simulink model "SE"  (R2019b)
settings: Solver=FixedStepDiscrete  StartTime=0.0  StopTime=stop_time  RelTol=1e-3
InitFcn:
  | sm_callback_init
StopFcn:
  | sm_callback_stop
values from neighbouring files (symbols this model uses):
  mp = sm_stop_verify(mp)    [sm_callback_stop.m]
libraries: hdlsllib x6, simulink x3
settings Model: Creator=Ross  LastModifiedBy=wickh
settings DataIOCC: ReturnWorkspaceOutputs=off
settings OptimizationCC: BlockReduction=off  ConditionallyExecuteInputs=off  DefaultParameterBehavior=Inlined
settings DebuggingCC: ReadBeforeWriteMsg=DisableAll  WriteAfterWriteMsg=DisableAll  WriteAfterReadMsg=DisableAll  AlgebraicLoopMsg=error  MultiTaskDSMMsg=none  SingleTaskRateTransMsg=error  PregeneratedLibrarySubsystemCodeDiagnostic=none  ArithmeticOperatorsInVariantConditions=warning
settings HardwareCC: ProdBitPerPointer=32  ProdBitPerSizeT=32  ProdBitPerPtrDiffT=32  ProdLargestAtomicFloat=None  ProdIntDivRoundTo=Undefined  ProdEndianess=Unspecified  ProdWordSize=32  ProdHWDeviceType=ASIC/FPGA->ASIC/FPGA  TargetBitPerPointer=64  TargetBitPerSizeT=64  TargetBitPerPtrDiffT=64  TargetLongLongMode=on  TargetIntDivRoundTo=Zero  TargetEndianess=LittleEndian  TargetWordSize=64  TargetHWDeviceType=Custom Processor->MATLAB Host Computer  ProdEqTarget=off
settings ModelReferenceCC: UpdateModelReferenceTargets=IfOutOfDate
settings SFSimCC: SFSimEcho=off  SimUseLocalCustomCode=off  CustomCodeUndefinedFunction=UseInterfaceOnly
settings RTWCC: RTWUseLocalCustomCode=off

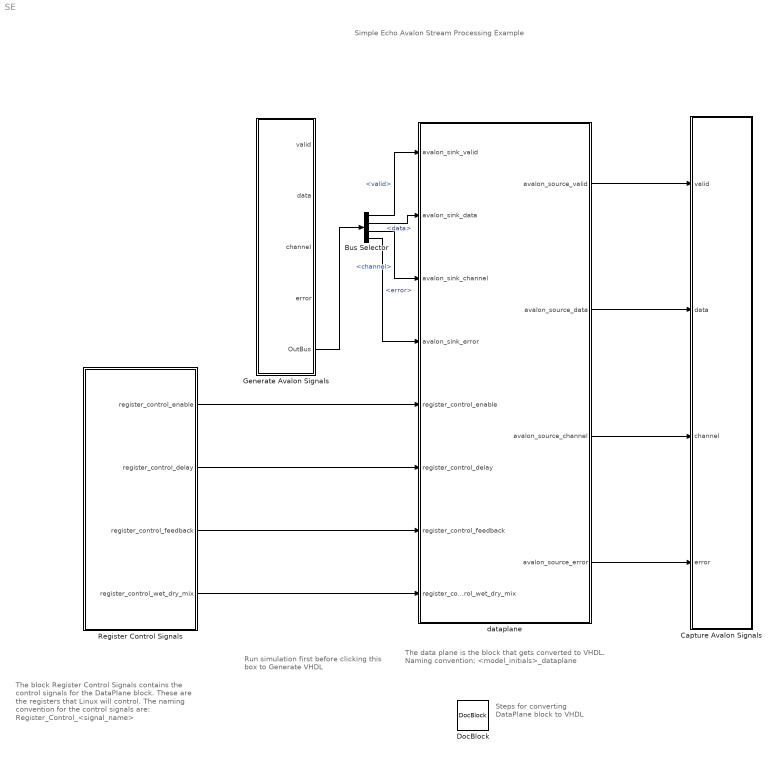
== system SE ==
  note: The data plane is the block that gets converted to VHDL. Naming convention: <model_initials>_dataplane
  note: Steps for converting
      | DataPlane block
      | to VHDL
  note: Simple Echo
      | Avalon Stream Processing Example
  note: Run simulation first
      | before clicking this box to
      | Generate VHDL
  note: The block Register Control Signals contains
      | the control signals for the DataPlane block.
      | These are the registers that Linux will control.
      | The naming convention for the control
      | signals are:  Register_Control_<signal_name>
  Bus Selector : BusSelector  OutputSignals=Avalon.valid,Avalon.data,Avalon.channel,Avalon.error
  Capture Avalon Signals : Subsystem
  DocBlock : simulink/Model-Wide Utilities/DocBlock  DocumentType=HTML
  Generate Avalon Signals : Subsystem
  Register Control Signals : Subsystem
  dataplane : Subsystem  TreatAsAtomicUnit=on
  wires:
  dataplane/2(avalon_source_data) -> Capture Avalon Signals/2(data)
  dataplane/1(avalon_source_valid) -> Capture Avalon Signals/1(valid)
  dataplane/3(avalon_source_channel) -> Capture Avalon Signals/3(channel)
  dataplane/4(avalon_source_error) -> Capture Avalon Signals/4(error)
  Register Control Signals/2(register_control_delay) -> dataplane/6(register_control_delay)
  Register Control Signals/1(register_control_enable) -> dataplane/5(register_control_enable)
  Register Control Signals/4(register_control_wet_dry_mix) -> dataplane/8(register_control_wet_dry_mix)
  Register Control Signals/3(register_control_feedback) -> dataplane/7(register_control_feedback)
  Generate Avalon Signals/5(OutBus) -> Bus Selector/1
  Bus Selector/1 -> dataplane/1(avalon_sink_valid)  "<valid>"
  Bus Selector/2 -> dataplane/2(avalon_sink_data)  "<data>"
  Bus Selector/3 -> dataplane/3(avalon_sink_channel)  "<channel>"
  Bus Selector/4 -> dataplane/4(avalon_sink_error)  "<error>"

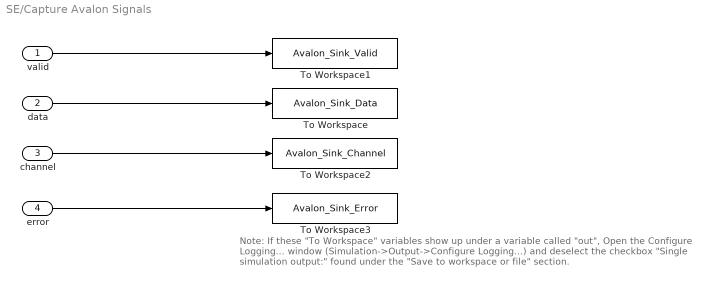
== system SE/Capture Avalon Signals ==
  note: Note:  If these "To Workspace" variables show up under a variable called "out",
      | Open the Configure Logging... window (Simulation->Output->Configure Logging...)
      | and deselect the checkbox "Single simulation output:" found under the "Save to workspace or file" section.
  valid : Inport
  data : Inport  Port=2
  channel : Inport  Port=3
  error : Inport  Port=4
  To Workspace : ToWorkspace  VariableName=Avalon_Sink_Data  SaveFormat=Timeseries  SampleTime=-1
  To Workspace1 : ToWorkspace  VariableName=Avalon_Sink_Valid  SaveFormat=Timeseries  SampleTime=-1
  To Workspace2 : ToWorkspace  VariableName=Avalon_Sink_Channel  SaveFormat=Timeseries  SampleTime=-1
  To Workspace3 : ToWorkspace  VariableName=Avalon_Sink_Error  SaveFormat=Timeseries  SampleTime=-1
  wires:
  data/1 -> To Workspace/1
  valid/1 -> To Workspace1/1
  error/1 -> To Workspace3/1
  channel/1 -> To Workspace2/1

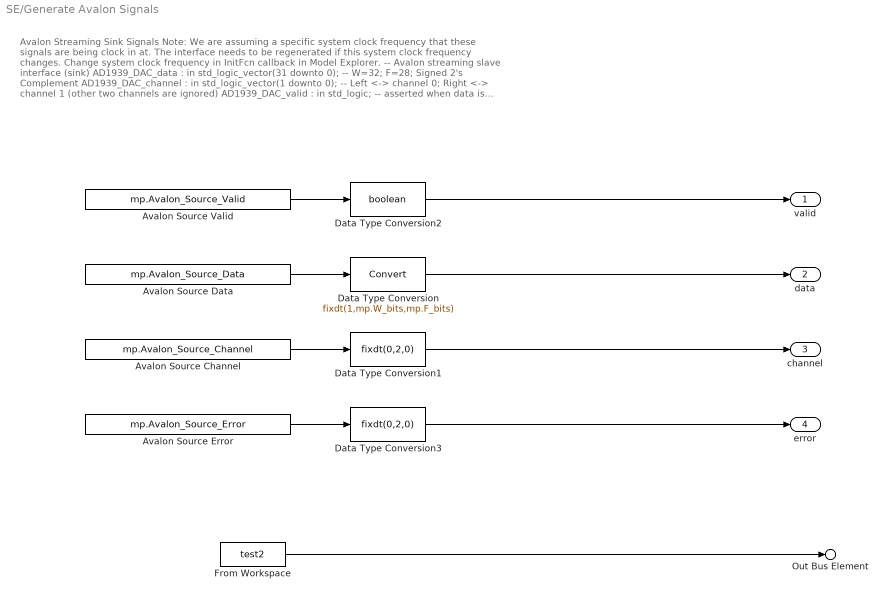
== system SE/Generate Avalon Signals ==
  note: Avalon Streaming Sink Signals
      | Note: We are assuming a specific system clock frequency that these signals are being clock in at.
      | The interface needs to be regenerated if this system clock frequency changes. Change system clock frequency in InitFcn callback in Model Explorer.
      |
      | -- Avalon streaming slave interface (sink)
      | AD1939_DAC_data : in std_logic_vector(31 downto 0); -- W=32; F=28; Signed 2's Complement
      | AD1939_DAC_channel : in std_logic_vector(1 downto 0); -- Left <-> channel 0; Right <-> channel 1 (other two channels are ignored)
      | AD1939_DAC_valid : in std_logic; -- asserted when data is valid
      | AD1939_DAC_error : in std_logic_vector(1 downto 0) -- error channel is ignored, assumed to be error free at this point
      |
      | For more information on the data-channel-valid protocol, s ee chapter 5 in Intel's Avalon Interfaced Specification (p. 40) at https://www.intel.com/content/dam/www/programmable/us/en/pdfs/literature/manual/mnl_avalon_spec.pdf
  Avalon Source Channel : FromWorkspace  VariableName=mp.Avalon_Source_Channel  OutDataTypeStr=double  SampleTime=mp.Ts_system
  "Avalon Source Data " : FromWorkspace  VariableName=mp.Avalon_Source_Data  OutDataTypeStr=double  SampleTime=mp.Ts_system
  Avalon Source Error : FromWorkspace  VariableName=mp.Avalon_Source_Error  OutDataTypeStr=double  SampleTime=mp.Ts_system
  Avalon Source Valid : FromWorkspace  VariableName=mp.Avalon_Source_Valid  OutDataTypeStr=double  SampleTime=mp.Ts_system
  Data Type Conversion : DataTypeConversion  OutDataTypeStr=fixdt(1,mp.W_bits,mp.F_bits)
  Data Type Conversion1 : DataTypeConversion  OutDataTypeStr=fixdt(0,2,0)
  Data Type Conversion2 : DataTypeConversion  OutDataTypeStr=boolean
  Data Type Conversion3 : DataTypeConversion  OutDataTypeStr=fixdt(0,2,0)
  From Workspace : FromWorkspace  VariableName=test2  OutDataTypeStr=Bus: AvalonBus  SampleTime=0
  valid : Outport  VectorParamsAs1DForOutWhenUnconnected=off
  data : Outport  Port=2  VectorParamsAs1DForOutWhenUnconnected=off
  channel : Outport  Port=3  VectorParamsAs1DForOutWhenUnconnected=off
  error : Outport  Port=4  VectorParamsAs1DForOutWhenUnconnected=off
  Out Bus Element : Outport  Port=5  PortName=OutBus  Element=Avalon
  wires:
  Data Type Conversion1/1 -> channel/1
  Data Type Conversion2/1 -> valid/1
  Avalon Source Error/1 -> Data Type Conversion3/1
  Data Type Conversion/1 -> data/1
  Avalon Source Valid/1 -> Data Type Conversion2/1
  Data Type Conversion3/1 -> error/1
  Avalon Source Channel/1 -> Data Type Conversion1/1
  "Avalon Source Data "/1 -> Data Type Conversion/1
  From Workspace/1 -> Out Bus Element/1

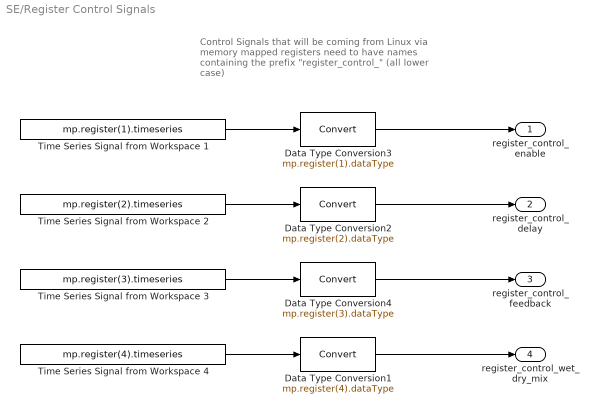
== system SE/Register Control Signals ==
  note: Control Signals that will be coming from Linux via
      | memory mapped registers need to have names
      | containing the prefix "register_control_"
      | (all lower case)
  Data Type Conversion1 : DataTypeConversion  OutDataTypeStr=mp.register(4).dataType
  Data Type Conversion2 : DataTypeConversion  OutDataTypeStr=mp.register(2).dataType
  Data Type Conversion3 : DataTypeConversion  OutDataTypeStr=mp.register(1).dataType
  Data Type Conversion4 : DataTypeConversion  OutDataTypeStr=mp.register(3).dataType
  Time Series Signal from Workspace 1 : FromWorkspace  VariableName=mp.register(1).timeseries  OutDataTypeStr=double  SampleTime=mp.Ts_system
  Time Series Signal from Workspace 2 : FromWorkspace  VariableName=mp.register(2).timeseries  OutDataTypeStr=double  SampleTime=mp.Ts_system
  Time Series Signal from Workspace 3 : FromWorkspace  VariableName=mp.register(3).timeseries  OutDataTypeStr=double  SampleTime=mp.Ts_system
  Time Series Signal from Workspace 4 : FromWorkspace  VariableName=mp.register(4).timeseries  OutDataTypeStr=double  SampleTime=mp.Ts_system
  register_control_enable : Outport  VectorParamsAs1DForOutWhenUnconnected=off
  register_control_delay : Outport  Port=2  VectorParamsAs1DForOutWhenUnconnected=off
  register_control_feedback : Outport  Port=3  VectorParamsAs1DForOutWhenUnconnected=off
  register_control_wet_dry_mix : Outport  Port=4  VectorParamsAs1DForOutWhenUnconnected=off
  wires:
  Time Series Signal from Workspace 2/1 -> Data Type Conversion2/1
  Data Type Conversion2/1 -> register_control_delay/1
  Time Series Signal from Workspace 1/1 -> Data Type Conversion3/1
  Data Type Conversion3/1 -> register_control_enable/1
  Time Series Signal from Workspace 4/1 -> Data Type Conversion1/1
  Data Type Conversion1/1 -> register_control_wet_dry_mix/1
  Data Type Conversion4/1 -> register_control_feedback/1
  Time Series Signal from Workspace 3/1 -> Data Type Conversion4/1

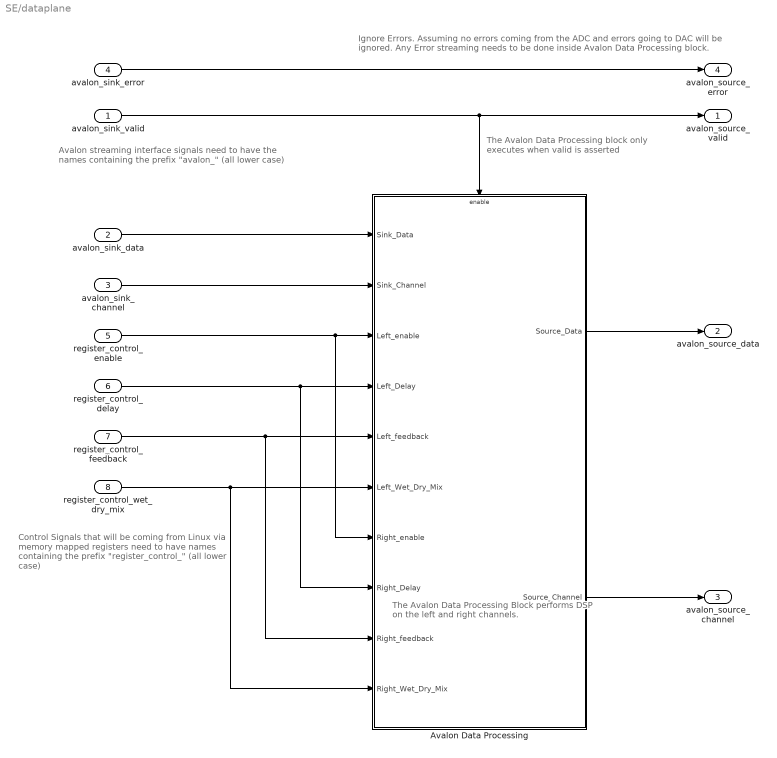
== system SE/dataplane ==
  note: Control Signals that will be coming from Linux via
      | memory mapped registers need to have names
      | containing the prefix "register_control_"
      | (all lower case)
  note: The Avalon Data Processing Block
      | performs DSP on the left and right channels.
  note: The Avalon Data Processing block
      | only executes when valid is asserted
  note: Ignore Errors.
      | Assuming no errors coming from the ADC and errors going to DAC will be ignored.
      | Any Error streaming needs to be done inside Avalon Data Processing block.
  note: Avalon streaming interface signals need to have the
      | names containing the prefix "avalon_"
      | (all lower case)
  avalon_sink_valid : Inport
  avalon_sink_data : Inport  Port=2
  avalon_sink_channel : Inport  Port=3
  avalon_sink_error : Inport  Port=4
  register_control_enable : Inport  Port=5
  register_control_delay : Inport  Port=6
  register_control_feedback : Inport  Port=7
  register_control_wet_dry_mix : Inport  Port=8
  Avalon Data Processing : Subsystem  TreatAsAtomicUnit=on
  avalon_source_valid : Outport  VectorParamsAs1DForOutWhenUnconnected=off
  avalon_source_data : Outport  Port=2  VectorParamsAs1DForOutWhenUnconnected=off
  avalon_source_channel : Outport  Port=3  VectorParamsAs1DForOutWhenUnconnected=off
  avalon_source_error : Outport  Port=4  VectorParamsAs1DForOutWhenUnconnected=off
  wires:
  avalon_sink_channel/1 -> Avalon Data Processing/2(Sink_Channel)
  avalon_sink_error/1 -> avalon_source_error/1
  Avalon Data Processing/1(Source_Data) -> avalon_source_data/1
  avalon_sink_valid/1 -> avalon_source_valid/1, Avalon Data Processing/Enable
  avalon_sink_data/1 -> Avalon Data Processing/1(Sink_Data)
  Avalon Data Processing/2(Source_Channel) -> avalon_source_channel/1
  register_control_delay/1 -> Avalon Data Processing/8(Right_Delay), Avalon Data Processing/4(Left_Delay)
  register_control_enable/1 -> Avalon Data Processing/7(Right_enable), Avalon Data Processing/3(Left_enable)
  register_control_wet_dry_mix/1 -> Avalon Data Processing/6(Left_Wet_Dry_Mix), Avalon Data Processing/10(Right_Wet_Dry_Mix)
  register_control_feedback/1 -> Avalon Data Processing/9(Right_feedback), Avalon Data Processing/5(Left_feedback)

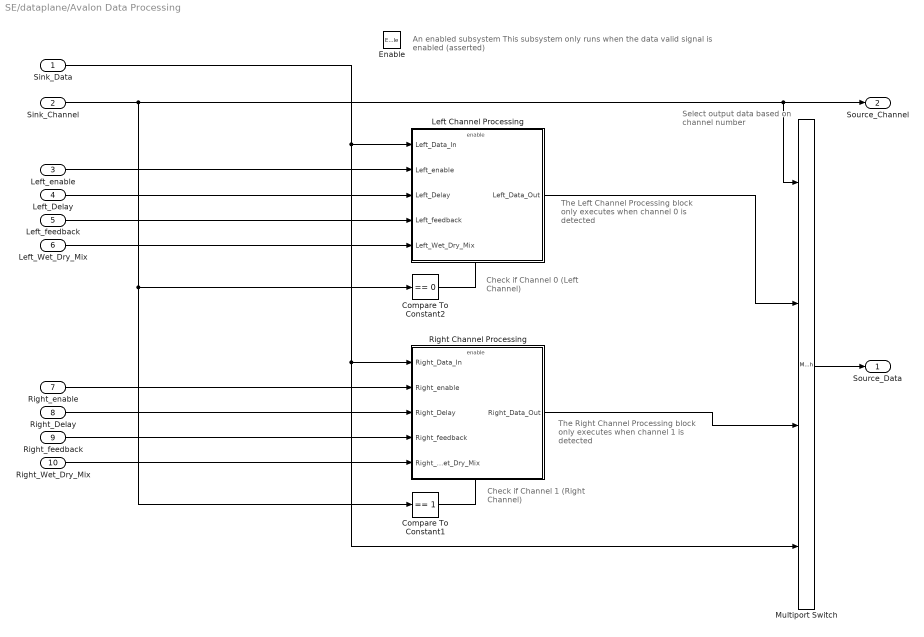
== system SE/dataplane/Avalon Data Processing ==
  note: Select output data
      | based on channel number
  note: Check if Channel 0
      | (Left Channel)
  note: The Left Channel Processing block
      | only executes when channel 0
      | is detected
  note: The Right Channel Processing block
      | only executes when channel 1
      | is detected
  note: Check if Channel 1
      | (Right Channel)
  note: An enabled subsystem
      | This subsystem only runs when the data valid signal is enabled (asserted)
  Sink_Data : Inport
  Sink_Channel : Inport  Port=2
  Left_enable : Inport  Port=3
  Left_Delay : Inport  Port=4
  Left_feedback : Inport  Port=5
  Left_Wet_Dry_Mix : Inport  Port=6
  Right_enable : Inport  Port=7
  Right_Delay : Inport  Port=8
  Right_feedback : Inport  Port=9
  Right_Wet_Dry_Mix : Inport  Port=10
  Enable : EnablePort
  Compare To Constant1 : simulink/Logic and Bit Operations/Compare To Constant  relop===  const=1  OutDataTypeStr=boolean
  Compare To Constant2 : simulink/Logic and Bit Operations/Compare To Constant  relop===  const=0  OutDataTypeStr=boolean
  Left Channel Processing : Subsystem  TreatAsAtomicUnit=on
  Multiport Switch : MultiPortSwitch  DataPortOrder=Zero-based contiguous  zeroidx=on
  Right Channel Processing : Subsystem  TreatAsAtomicUnit=on
  Source_Data : Outport  InitialOutput=0  VectorParamsAs1DForOutWhenUnconnected=off
  Source_Channel : Outport  Port=2  InitialOutput=0  VectorParamsAs1DForOutWhenUnconnected=off
  wires:
  Sink_Channel/1 -> Compare To Constant1/1, Compare To Constant2/1, Source_Channel/1, Multiport Switch/1
  Compare To Constant2/1 -> Left Channel Processing/Enable
  Compare To Constant1/1 -> Right Channel Processing/Enable
  Sink_Data/1 -> Multiport Switch/4, Right Channel Processing/1(Right_Data_In), Left Channel Processing/1(Left_Data_In)
  Left Channel Processing/1("Left_Data_Out ") -> Multiport Switch/2
  Right Channel Processing/1("Right_Data_Out ") -> Multiport Switch/3
  Multiport Switch/1 -> Source_Data/1
  Left_Delay/1 -> Left Channel Processing/3(Left_Delay)
  Right_Delay/1 -> Right Channel Processing/3(Right_Delay)
  Left_enable/1 -> Left Channel Processing/2(Left_enable)
  Right_enable/1 -> Right Channel Processing/2(Right_enable)
  Left_Wet_Dry_Mix/1 -> Left Channel Processing/5(Left_Wet_Dry_Mix)
  Right_Wet_Dry_Mix/1 -> Right Channel Processing/5(Right_Wet_Dry_Mix)
  Left_feedback/1 -> Left Channel Processing/4(Left_feedback)
  Right_feedback/1 -> Right Channel Processing/4(Right_feedback)

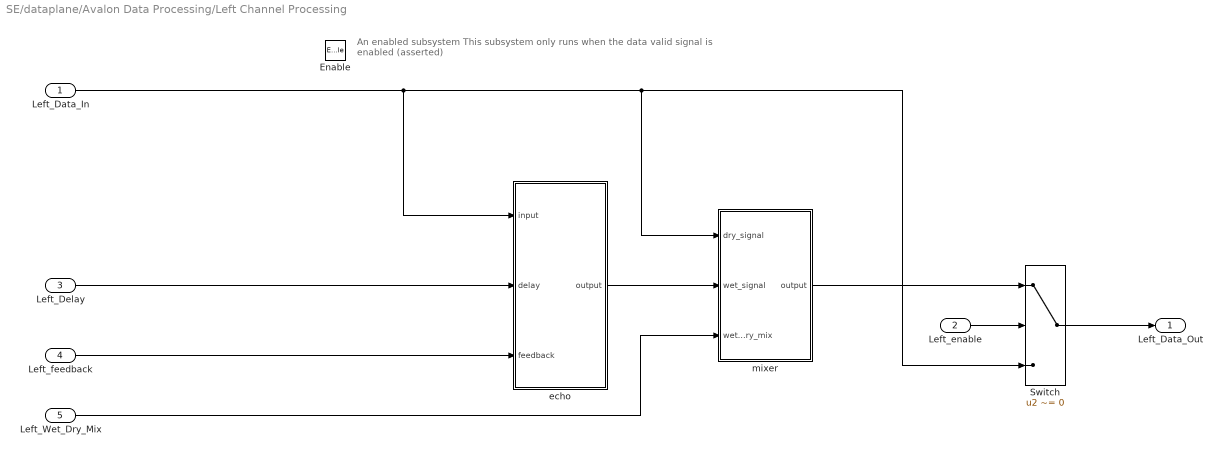
== system SE/dataplane/Avalon Data Processing/Left Channel Processing ==
  note: An enabled subsystem
      | This subsystem only runs when the data valid signal is enabled (asserted)
  Left_Data_In : Inport
  Left_enable : Inport  Port=2
  Left_Delay : Inport  Port=3
  Left_feedback : Inport  Port=4
  Left_Wet_Dry_Mix : Inport  Port=5
  Enable : EnablePort
  Switch : Switch  Criteria=u2 ~= 0
  echo : Subsystem
  mixer : Subsystem
  "Left_Data_Out " : Outport  InitialOutput=0  VectorParamsAs1DForOutWhenUnconnected=off
  wires:
  Left_Data_In/1 -> echo/1(input), mixer/1(dry_signal), Switch/3
  Switch/1 -> "Left_Data_Out "/1
  Left_enable/1 -> Switch/2
  echo/1(output) -> mixer/2(wet_signal)
  Left_Wet_Dry_Mix/1 -> mixer/3(wet_dry_mix)
  Left_Delay/1 -> echo/2(delay)
  Left_feedback/1 -> echo/3(feedback)
  mixer/1(output) -> Switch/1

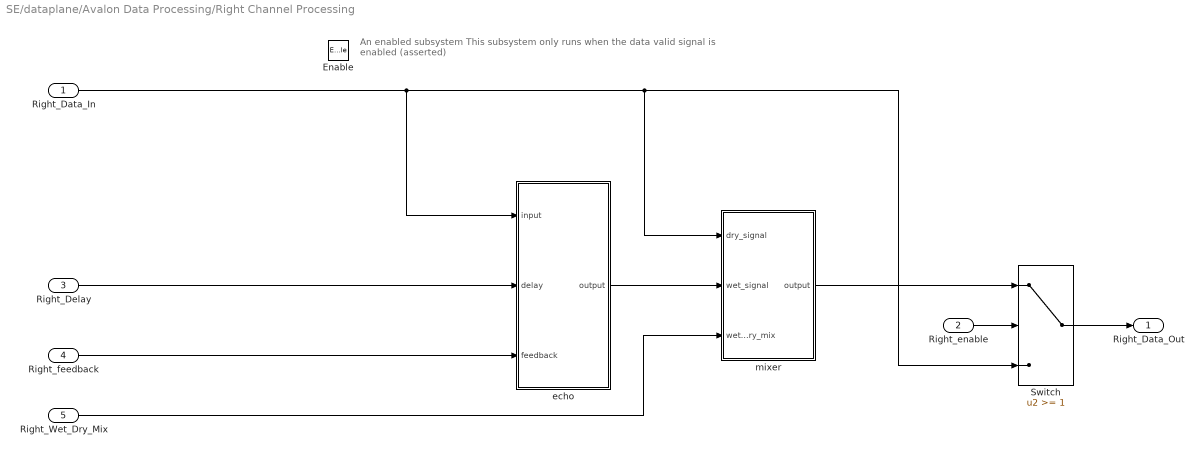
== system SE/dataplane/Avalon Data Processing/Right Channel Processing ==
  note: An enabled subsystem
      | This subsystem only runs when the data valid signal is enabled (asserted)
  Right_Data_In : Inport
  Right_enable : Inport  Port=2
  Right_Delay : Inport  Port=3
  Right_feedback : Inport  Port=4
  Right_Wet_Dry_Mix : Inport  Port=5
  Enable : EnablePort
  Switch : Switch  Threshold=1
  echo : Subsystem
  mixer : Subsystem
  "Right_Data_Out " : Outport  InitialOutput=0  VectorParamsAs1DForOutWhenUnconnected=off
  wires:
  Right_Data_In/1 -> echo/1(input), Switch/3, mixer/1(dry_signal)
  Switch/1 -> "Right_Data_Out "/1
  Right_enable/1 -> Switch/2
  echo/1(output) -> mixer/2(wet_signal)
  Right_Wet_Dry_Mix/1 -> mixer/3(wet_dry_mix)
  Right_Delay/1 -> echo/2(delay)
  Right_feedback/1 -> echo/3(feedback)
  mixer/1(output) -> Switch/1

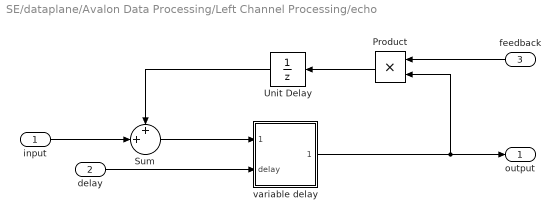
== system SE/dataplane/Avalon Data Processing/Left Channel Processing/echo ==
  input : Inport
  delay : Inport  Port=2
  feedback : Inport  Port=3
  Product : Product  OutDataTypeStr=fixdt(1,mp.W_bits,mp.F_bits)
  Sum : Sum  Inputs=++|
  Unit Delay : UnitDelay  SampleTime=-1  HasFrameUpgradeWarning=on
  variable delay : Subsystem
  output : Outport  VectorParamsAs1DForOutWhenUnconnected=off
  wires:
  delay/1 -> variable delay/2(delay)
  input/1 -> Sum/2
  Sum/1 -> variable delay/1(data_in)
  Unit Delay/1 -> Sum/1
  Product/1 -> Unit Delay/1
  variable delay/1(data_out) -> output/1, Product/2
  feedback/1 -> Product/1

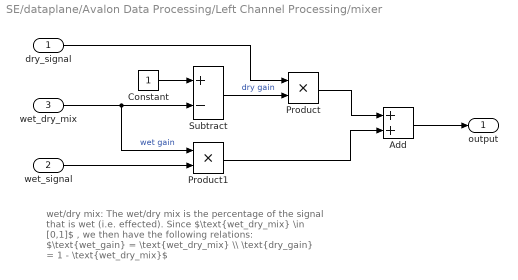
== system SE/dataplane/Avalon Data Processing/Left Channel Processing/mixer ==
  note: wet/dry mix:
      | The wet/dry mix is the percentage of the signal that is wet (i.e. effected).
      |
      | Since $\text{wet_dry_mix} \in [0,1]$ , we then have the following relations:
      | $\text{wet_gain} = \text{wet_dry_mix} \\ \text{dry_gain} = 1 - \text{wet_dry_mix}$
  dry_signal : Inport
  wet_signal : Inport  Port=2
  wet_dry_mix : Inport  Port=3
  Add : Sum  OutDataTypeStr=fixdt(1,mp.W_bits,mp.F_bits)
  Constant : Constant  OutDataTypeStr=Inherit: Inherit via back propagation  SampleTime=-1
  Product : Product
  Product1 : Product
  Subtract : Sum  Inputs=+-  InputSameDT=on  OutDataTypeStr=Inherit: Same as first input
  output : Outport  VectorParamsAs1DForOutWhenUnconnected=off
  wires:
  wet_dry_mix/1 -> Product1/1, Subtract/2  "wet gain"
  Product/1 -> Add/1
  wet_signal/1 -> Product1/2
  Product1/1 -> Add/2
  Subtract/1 -> Product/2  "dry gain"
  dry_signal/1 -> Product/1
  Add/1 -> output/1
  Constant/1 -> Subtract/1

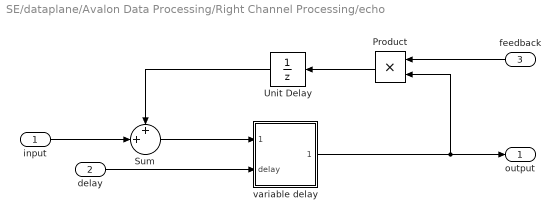
== system SE/dataplane/Avalon Data Processing/Right Channel Processing/echo ==
  input : Inport
  delay : Inport  Port=2
  feedback : Inport  Port=3
  Product : Product  OutDataTypeStr=fixdt(1,mp.W_bits,mp.F_bits)
  Sum : Sum  Inputs=++|
  Unit Delay : UnitDelay  SampleTime=-1  HasFrameUpgradeWarning=on
  variable delay : Subsystem
  output : Outport  VectorParamsAs1DForOutWhenUnconnected=off
  wires:
  Sum/1 -> variable delay/1(data_in)
  Unit Delay/1 -> Sum/1
  input/1 -> Sum/2
  delay/1 -> variable delay/2(delay)
  feedback/1 -> Product/1
  Product/1 -> Unit Delay/1
  variable delay/1(data_out) -> output/1, Product/2

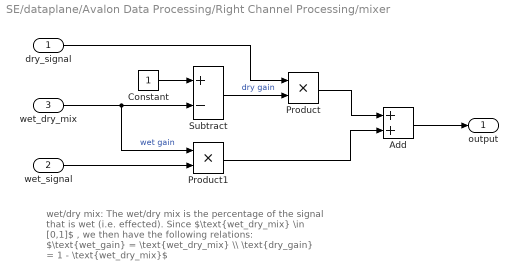
== system SE/dataplane/Avalon Data Processing/Right Channel Processing/mixer ==
  note: wet/dry mix:
      | The wet/dry mix is the percentage of the signal that is wet (i.e. effected).
      |
      | Since $\text{wet_dry_mix} \in [0,1]$ , we then have the following relations:
      | $\text{wet_gain} = \text{wet_dry_mix} \\ \text{dry_gain} = 1 - \text{wet_dry_mix}$
  dry_signal : Inport
  wet_signal : Inport  Port=2
  wet_dry_mix : Inport  Port=3
  Add : Sum  OutDataTypeStr=fixdt(1,mp.W_bits,mp.F_bits)
  Constant : Constant  OutDataTypeStr=Inherit: Inherit via back propagation  SampleTime=-1
  Product : Product
  Product1 : Product
  Subtract : Sum  Inputs=+-  InputSameDT=on  OutDataTypeStr=Inherit: Same as first input
  output : Outport  VectorParamsAs1DForOutWhenUnconnected=off
  wires:
  Add/1 -> output/1
  Constant/1 -> Subtract/1
  wet_dry_mix/1 -> Product1/1, Subtract/2  "wet gain"
  Product/1 -> Add/1
  Product1/1 -> Add/2
  wet_signal/1 -> Product1/2
  dry_signal/1 -> Product/1
  Subtract/1 -> Product/2  "dry gain"

== system SE/dataplane/Avalon Data Processing/Left Channel Processing/echo/variable delay ==
  data_in : Inport
  delay : Inport  Port=2
  Constant : Constant  OutDataTypeStr=Inherit: Inherit via back propagation  SampleTime=-1
  Simple Dual Port RAM : hdlsllib/HDL RAMs/Simple Dual Port RAM  ram_size=mp.dpram_addr_size
      settings: SourceProductName=Simulink  SourceProductBaseCode=SL
  read address generator : Subsystem
  write address generator : hdlsllib/Sources/HDL Counter  CountType=Count limited  CountInit=0  CountStep=1  CountMax=2^mp.dpram_addr_size - 1  CountFromType=Initial value  CountFrom=0  CountResetPort=off  CountLoadPort=off  CountEnbPort=off  CountDirPort=off  CountDataType=Unsigned  CountWordLen=mp.dpram_addr_size  CountFracLen=0  CountSampTime=mp.Ts_system
      settings: SourceProductName=Simulink
  data_out : Outport  VectorParamsAs1DForOutWhenUnconnected=off
  wires:
  Constant/1 -> Simple Dual Port RAM/3
  Simple Dual Port RAM/1 -> data_out/1
  write address generator/1 -> Simple Dual Port RAM/2, read address generator/2(write_addr)
  data_in/1 -> Simple Dual Port RAM/1
  read address generator/1(read_addr) -> Simple Dual Port RAM/4
  delay/1 -> read address generator/1(delay)

== system SE/dataplane/Avalon Data Processing/Right Channel Processing/echo/variable delay ==
  data_in : Inport
  delay : Inport  Port=2
  Constant : Constant  OutDataTypeStr=Inherit: Inherit via back propagation  SampleTime=-1
  Simple Dual Port RAM : hdlsllib/HDL RAMs/Simple Dual Port RAM  ram_size=mp.dpram_addr_size
      settings: SourceProductName=Simulink  SourceProductBaseCode=SL
  read address generator : Subsystem
  write address generator : hdlsllib/Sources/HDL Counter  CountType=Count limited  CountInit=0  CountStep=1  CountMax=2^mp.dpram_addr_size - 1  CountFromType=Initial value  CountFrom=0  CountResetPort=off  CountLoadPort=off  CountEnbPort=off  CountDirPort=off  CountDataType=Unsigned  CountWordLen=mp.dpram_addr_size  CountFracLen=0  CountSampTime=mp.Ts_system
      settings: SourceProductName=Simulink
  data_out : Outport  VectorParamsAs1DForOutWhenUnconnected=off
  wires:
  Constant/1 -> Simple Dual Port RAM/3
  Simple Dual Port RAM/1 -> data_out/1
  write address generator/1 -> Simple Dual Port RAM/2, read address generator/2(write_addr)
  data_in/1 -> Simple Dual Port RAM/1
  read address generator/1(read_addr) -> Simple Dual Port RAM/4
  delay/1 -> read address generator/1(delay)

== system SE/dataplane/Avalon Data Processing/Left Channel Processing/echo/variable delay/read address generator ==
  note: read address should trail the write address by "delay" number of samples.
      |
      | wrap on overflow is the desired behavior
  note: When the delay value changes, we reload the counter with the new read address value
  note: check if delay changed
  delay : Inport
  write_addr : Inport  Port=2
  Constant : Constant  Value=2  OutDataTypeStr=Inherit: Inherit via back propagation  SampleTime=-1
  Memory : Memory  InheritSampleTime=on
  Relational Operator : RelationalOperator  Operator=~=  OutDataTypeStr=boolean  RndMeth=Nearest
  Subtract : Sum  Inputs=-++  InputSameDT=on  OutDataTypeStr=Inherit: Same as first input
  read address counter : hdlsllib/Sources/HDL Counter  CountType=Count limited  CountInit=0  CountStep=1  CountMax=2^mp.dpram_addr_size - 1  CountFromType=Initial value  CountFrom=0  CountResetPort=off  CountLoadPort=on  CountEnbPort=off  CountDirPort=off  CountDataType=Unsigned  CountWordLen=mp.dpram_addr_size  CountFracLen=0  CountSampTime=-1
      settings: SourceProductName=Simulink
  read_addr : Outport  VectorParamsAs1DForOutWhenUnconnected=off
  wires:
  read address counter/1 -> read_addr/1
  delay/1 -> Memory/1, Relational Operator/2, Subtract/1
  Memory/1 -> Relational Operator/1
  Relational Operator/1 -> read address counter/1  "delay_changed"
  write_addr/1 -> Subtract/2
  Subtract/1 -> read address counter/2
  Constant/1 -> Subtract/3

== system SE/dataplane/Avalon Data Processing/Right Channel Processing/echo/variable delay/read address generator ==
  note: read address should trail the write address by "delay" number of samples.
      |
      | wrap on overflow is the desired behavior
  note: When the delay value changes, we reload the counter with the new read address value
  note: check if delay changed
  delay : Inport
  write_addr : Inport  Port=2
  Constant : Constant  Value=2  OutDataTypeStr=Inherit: Inherit via back propagation  SampleTime=-1
  Memory : Memory  InheritSampleTime=on
  Relational Operator : RelationalOperator  Operator=~=  OutDataTypeStr=boolean  RndMeth=Nearest
  Subtract : Sum  Inputs=-++  InputSameDT=on  OutDataTypeStr=Inherit: Same as first input
  read address counter : hdlsllib/Sources/HDL Counter  CountType=Count limited  CountInit=0  CountStep=1  CountMax=2^mp.dpram_addr_size - 1  CountFromType=Initial value  CountFrom=0  CountResetPort=off  CountLoadPort=on  CountEnbPort=off  CountDirPort=off  CountDataType=Unsigned  CountWordLen=mp.dpram_addr_size  CountFracLen=0  CountSampTime=-1
      settings: SourceProductName=Simulink
  read_addr : Outport  VectorParamsAs1DForOutWhenUnconnected=off
  wires:
  read address counter/1 -> read_addr/1
  delay/1 -> Memory/1, Relational Operator/2, Subtract/1
  Memory/1 -> Relational Operator/1
  Relational Operator/1 -> read address counter/1  "delay_changed"
  write_addr/1 -> Subtract/2
  Subtract/1 -> read address counter/2
  Constant/1 -> Subtract/3
